simulink model "linmodel_eq1_discr_2018a"  (R2018a)
settings: Solver=VariableStepAuto  StartTime=0.0  StopTime=30  RelTol=1e-3
InitFcn:
  | lin_discr_model
undefined symbols (not defined in the file or in its folder): A_eq1_d, B_eq1_d, C_eq1_d, D_eq1_d, Discrete, Time, Ts
libraries: ctrlSharedLib x1
settings Model: Creator=jessi  LastModifiedBy=jessi
settings DataIOCC: ReturnWorkspaceOutputs=on
settings SFSimCC: SimUseLocalCustomCode=on
settings RTWCC: RTWUseLocalCustomCode=on

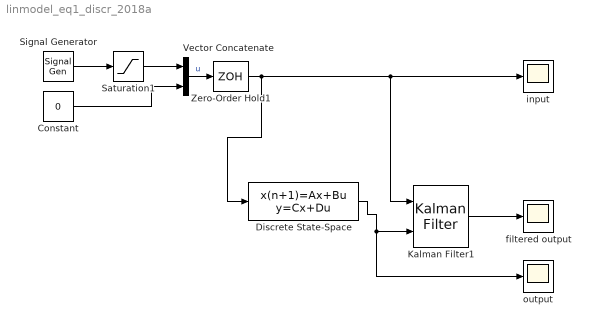
== system linmodel_eq1_discr_2018a ==
  Constant : Constant  Value=0
  Discrete State-Space : DiscreteStateSpace  A=A_eq1_d  B=B_eq1_d  C=C_eq1_d  D=D_eq1_d  InitialCondition=[pi;0;0;0]  SampleTime=Ts
  Kalman Filter1 : ctrlSharedLib/Kalman Filter  TimeDomain=Discrete-Time  UseCurrentEstimator=on  ModelSource=Individual A, B, C, D matrices  ModelSourceVariable=ss(0.95,1,1,0,1)  A=A_eq1_d  B=B_eq1_d  C=C_eq1_d  D=D_eq1_d  NumberOfStates=1  NumberOfInputs=1  NumberOfOutputs=1  InitialEstimateSource=Dialog  X0=[pi;0;0;0]  P0=10  UseK=off  UseGH=off  NumberOfProcessNoiseInputs=1  G=1  TimeInvariantG=on  H=0  TimeInvariantH=on  Q=0.05  TimeInvariantQ=on  R=1  TimeInvariantR=on  N=0  TimeInvariantN=on  AddInputPort=on  AddEnablePort=off  OutputEstimatedY=off  OutputP=off  Ts=Ts
      settings: SourceProductBaseCode=CT
  Saturation1 : Saturate  UpperLimit=1  LowerLimit=-1
  Signal Generator : SignalGenerator  WaveForm=square  Amplitude=0.3
  Vector Concatenate : Concatenate
  Zero-Order Hold1 : ZeroOrderHold  SampleTime=Ts
  filtered output : Scope
  input : Scope
  output : Scope
  wires:
  Constant/1 -> Vector Concatenate/2
  Vector Concatenate/1 -> Zero-Order Hold1/1  "u"
  Signal Generator/1 -> Saturation1/1
  Saturation1/1 -> Vector Concatenate/1
  Zero-Order Hold1/1 -> input/1, Kalman Filter1/1, Discrete State-Space/1
  Discrete State-Space/1 -> output/1, Kalman Filter1/2
  Kalman Filter1/1 -> filtered output/1
